simulink model "drugi"  (R2017b)
settings: Solver=VariableStepAuto  StartTime=0.0  StopTime=10.0  RelTol=1e-3
settings Model: Creator=USER  LastModifiedBy=USER

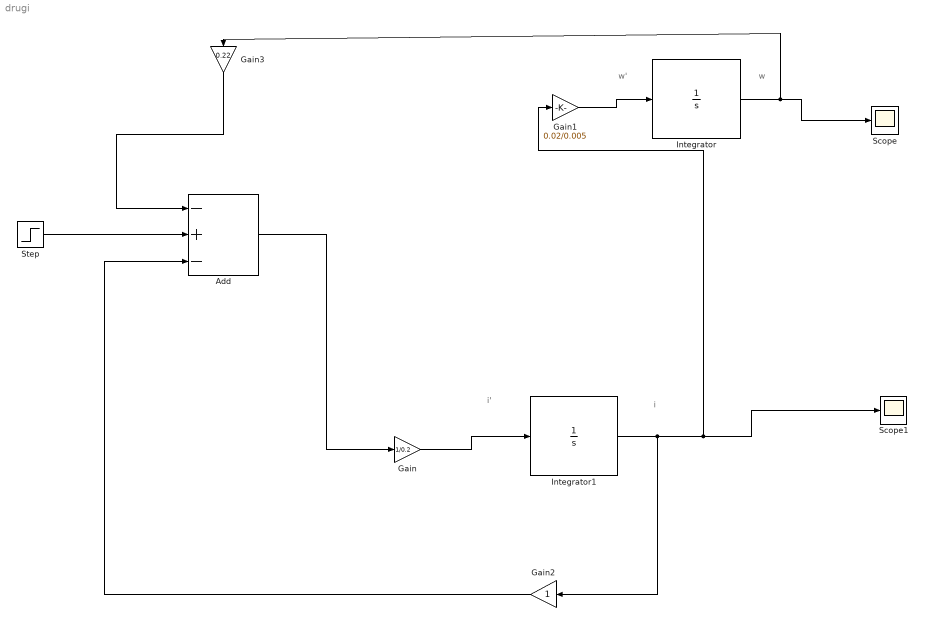
== system drugi ==
  note: w'
  note: w
  note: i'
  note: i
  Add : Sum  Inputs=-+-
  Gain : Gain  Gain=1/0.2
  Gain1 : Gain  Gain=0.02/0.005
  Gain2 : Gain
  Gain3 : Gain  Gain=0.22
  Integrator : Integrator
  Integrator1 : Integrator
  Scope : Scope
  Scope1 : Scope
  Step : Step  Time=0  SampleTime=0
  wires:
  Step/1 -> Add/2
  Gain/1 -> Integrator1/1
  Add/1 -> Gain/1
  Gain1/1 -> Integrator/1
  Integrator1/1 -> Gain2/1, Gain1/1, Scope1/1
  Integrator/1 -> Gain3/1, Scope/1
  Gain3/1 -> Add/1
  Gain2/1 -> Add/3
